simulink model "b"  (R2012b)
settings: Solver=ode45  StartTime=0.0  StopTime=10.0  RelTol=1e-3
values from neighbouring files (symbols this model uses):
  K_FACTOR = [137.465208994 137.065019157 135.864449646 135.664354728 137.565256453 140.366585312 145.268910814 152.872517717 162.9773111 164.27792807 166.178829795 167.979684062 ... (21 elements, 21x1)]    [torque_converter.mat]
  SPEED_RATIO = [0 0.1 0.2 0.3 0.4 0.5 0.6 0.7 0.8 0.81 0.82 0.83 ... (21 elements, 21x1)]    [torque_converter.mat]
  TORQUE_RATIO = [2.232 2.075 1.975 1.846 1.72 1.564 1.409 1.254 1.096 1.08 1.061 1.043 ... (21 elements, 21x1)]    [torque_converter.mat]
undefined symbols (not defined in the file or in its folder): magnitude
settings Model: Creator=ZhouHaoyu  LastModifiedBy=ZhouHaoyu
settings DataIOCC: ExternalInput=[t,N_engine,N_turbine]  LoadExternalInput=on

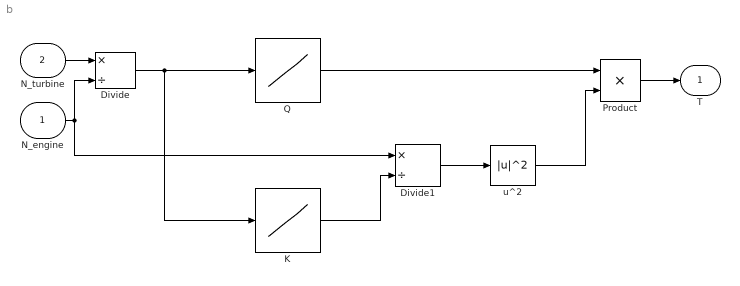
== system b ==
  N_engine : Inport
  N_turbine : Inport  Port=2
  Divide : Product  Inputs=*/
  Divide1 : Product  Inputs=*/
  K : Lookup_n-D  NumberOfTableDimensions=1  BreakpointsForDimension1=SPEED_RATIO  Table=K_FACTOR  RndMeth=Simplest  InputSameDT=on
  Product : Product  RndMeth=Zero
  Q : Lookup_n-D  NumberOfTableDimensions=1  BreakpointsForDimension1=SPEED_RATIO  Table=TORQUE_RATIO  RndMeth=Simplest  InputSameDT=on
  u^2 : Math  Operator=magnitude^2  SaturateOnIntegerOverflow=on
  T : Outport
  wires:
  N_engine/1 -> Divide1/1, Divide/2
  N_turbine/1 -> Divide/1
  Divide/1 -> K/1, Q/1
  K/1 -> Divide1/2
  Divide1/1 -> u^2/1
  u^2/1 -> Product/2
  Q/1 -> Product/1
  Product/1 -> T/1
